simulink model "uav_airframe"  (R2023b)
settings: Solver=ode45  StartTime=0  StopTime=500  RelTol=1e-4
undefined symbols (not defined in the file): b, c, C_D, C_l, C_L, C_m, C_n, C_Q, C_T, C_Y, D, F_b, i_0, K_Q, K_V, M_b, mass, p, R_motor, S, V_max
libraries: sharedtransform x2
settings Model: Creator=Victor  LastModifiedBy=Victor
settings DataIOCC: ExternalInput=getinputstruct(report30)  InitialState=getstatestruct(report30)  SaveOutput=off  SaveTime=off
settings DebuggingCC: MaxConsecutiveZCsMsg=warning

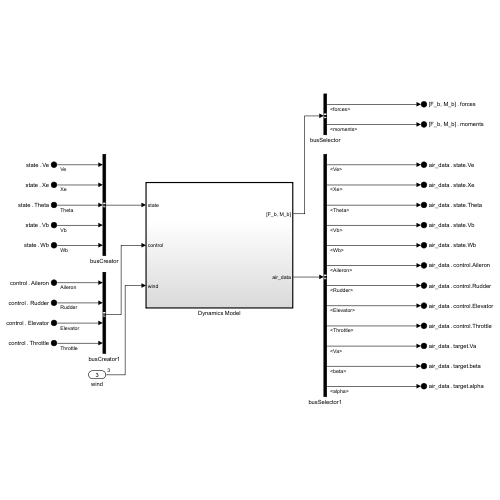
[thumbnail: Simulink's stored preview of the top-level diagram]
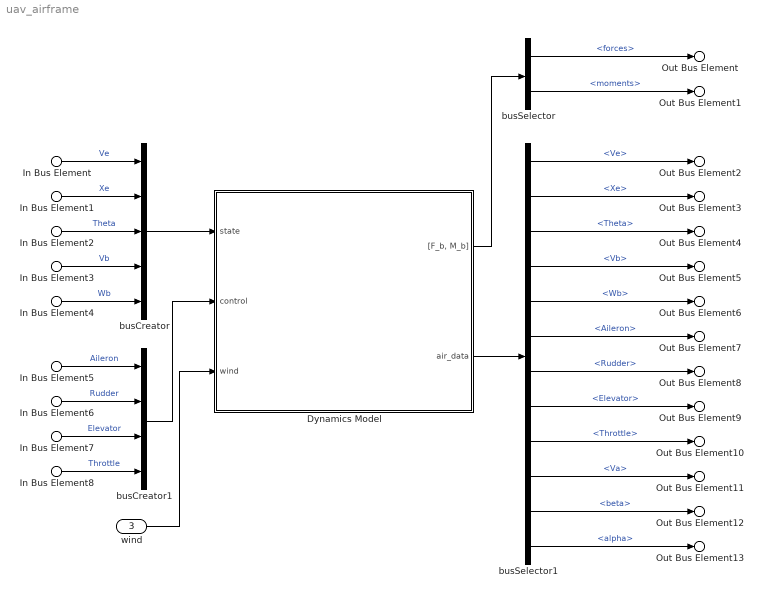
== system uav_airframe ==
  In Bus Element : Inport  PortName=state  Element=Ve
  In Bus Element1 : Inport  PortName=state  Element=Xe
  In Bus Element2 : Inport  PortName=state  Element=Theta
  In Bus Element3 : Inport  PortName=state  Element=Vb
  In Bus Element4 : Inport  PortName=state  Element=Wb
  In Bus Element5 : Inport  Port=2  PortName=control  Element=Aileron
  In Bus Element6 : Inport  Port=2  PortName=control  Element=Rudder
  In Bus Element7 : Inport  Port=2  PortName=control  Element=Elevator
  In Bus Element8 : Inport  Port=2  PortName=control  Element=Throttle
  wind : Inport  Port=3  OutDataTypeStr=double  PortDimensions=3
  Dynamics Model : Subsystem  TreatAsAtomicUnit=on
  busCreator : BusCreator  Inputs=5
  busCreator1 : BusCreator  Inputs=4
  busSelector : BusSelector  OutputSignals=forces,moments
  busSelector1 : BusSelector  OutputSignals=state.Ve,state.Xe,state.Theta,state.Vb,state.Wb,control.Aileron,control.Rudder,control.Elevator,control.Throttle,target.Va,target.beta,target.alpha
  Out Bus Element : Outport  PortName=[F_b, M_b]  Element=forces
  Out Bus Element1 : Outport  PortName=[F_b, M_b]  Element=moments
  Out Bus Element2 : Outport  Port=2  PortName=air_data  Element=state.Ve
  Out Bus Element3 : Outport  Port=2  PortName=air_data  Element=state.Xe
  Out Bus Element4 : Outport  Port=2  PortName=air_data  Element=state.Theta
  Out Bus Element5 : Outport  Port=2  PortName=air_data  Element=state.Vb
  Out Bus Element6 : Outport  Port=2  PortName=air_data  Element=state.Wb
  Out Bus Element7 : Outport  Port=2  PortName=air_data  Element=control.Aileron
  Out Bus Element8 : Outport  Port=2  PortName=air_data  Element=control.Rudder
  Out Bus Element9 : Outport  Port=2  PortName=air_data  Element=control.Elevator
  Out Bus Element10 : Outport  Port=2  PortName=air_data  Element=control.Throttle
  Out Bus Element11 : Outport  Port=2  PortName=air_data  Element=target.Va
  Out Bus Element12 : Outport  Port=2  PortName=air_data  Element=target.beta
  Out Bus Element13 : Outport  Port=2  PortName=air_data  Element=target.alpha
  wires:
  In Bus Element/1 -> busCreator/1  "Ve"
  In Bus Element1/1 -> busCreator/2  "Xe"
  In Bus Element5/1 -> busCreator1/1  "Aileron"
  In Bus Element2/1 -> busCreator/3  "Theta"
  In Bus Element6/1 -> busCreator1/2  "Rudder"
  In Bus Element3/1 -> busCreator/4  "Vb"
  In Bus Element7/1 -> busCreator1/3  "Elevator"
  In Bus Element4/1 -> busCreator/5  "Wb"
  In Bus Element8/1 -> busCreator1/4  "Throttle"
  busCreator/1 -> Dynamics Model/1(state)
  busCreator1/1 -> Dynamics Model/2(control)
  wind/1 -> Dynamics Model/3(wind)
  busSelector/2 -> Out Bus Element1/1  "<moments>"
  Dynamics Model/1("[F_b, M_b]") -> busSelector/1
  busSelector1/4 -> Out Bus Element5/1  "<Vb>"
  Dynamics Model/2(air_data) -> busSelector1/1
  busSelector/1 -> Out Bus Element/1  "<forces>"
  busSelector1/1 -> Out Bus Element2/1  "<Ve>"
  busSelector1/2 -> Out Bus Element3/1  "<Xe>"
  busSelector1/3 -> Out Bus Element4/1  "<Theta>"
  busSelector1/5 -> Out Bus Element6/1  "<Wb>"
  busSelector1/6 -> Out Bus Element7/1  "<Aileron>"
  busSelector1/7 -> Out Bus Element8/1  "<Rudder>"
  busSelector1/8 -> Out Bus Element9/1  "<Elevator>"
  busSelector1/9 -> Out Bus Element10/1  "<Throttle>"
  busSelector1/10 -> Out Bus Element11/1  "<Va>"
  busSelector1/11 -> Out Bus Element12/1  "<beta>"
  busSelector1/12 -> Out Bus Element13/1  "<alpha>"

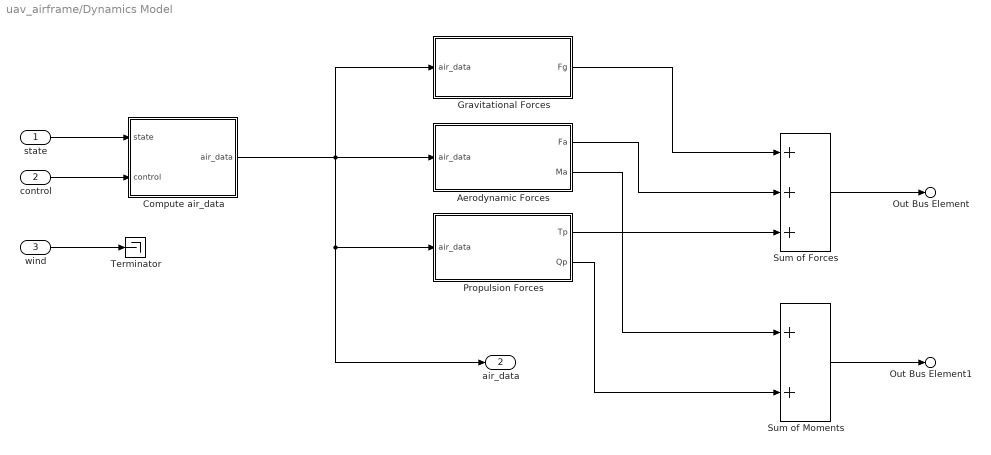
== system uav_airframe/Dynamics Model ==
  state : Inport
  control : Inport  Port=2
  wind : Inport  Port=3
  Aerodynamic Forces : Subsystem
  Compute air_data : Subsystem
  Gravitational Forces : Subsystem
  Propulsion Forces : Subsystem
  Sum of Forces : Sum  Inputs=+++
  Sum of Moments : Sum
  Terminator : Terminator
  Out Bus Element : Outport  PortName=[F_b, M_b]  Element=forces
  Out Bus Element1 : Outport  PortName=[F_b, M_b]  Element=moments
  air_data : Outport  Port=2
  wires:
  Propulsion Forces/2(Qp) -> Sum of Moments/2
  Propulsion Forces/1(Tp) -> Sum of Forces/3
  Compute air_data/1(air_data) -> Aerodynamic Forces/1(air_data), Gravitational Forces/1(air_data), air_data/1, Propulsion Forces/1(air_data)
  control/1 -> Compute air_data/2(control)
  state/1 -> Compute air_data/1(state)
  wind/1 -> Terminator/1
  Sum of Forces/1 -> Out Bus Element/1
  Sum of Moments/1 -> Out Bus Element1/1
  Gravitational Forces/1(Fg) -> Sum of Forces/1
  Aerodynamic Forces/1(Fa) -> Sum of Forces/2
  Aerodynamic Forces/2(Ma) -> Sum of Moments/1

== system uav_airframe/Dynamics Model/Aerodynamic Forces ==
  air_data : Inport
  Add : Sum
  Add1 : Sum
  Lateral Forces : Subsystem
  Longitudinal Forces : Subsystem
  Fa : Outport
  Ma : Outport  Port=2
  wires:
  air_data/1 -> Lateral Forces/1(air_data), Longitudinal Forces/1(air_data)
  Lateral Forces/1(faL_b) -> Add/1
  Longitudinal Forces/1(fa_b) -> Add/2
  Add/1 -> Fa/1
  Lateral Forces/2(MaL_b) -> Add1/1
  Longitudinal Forces/2(Ma_b) -> Add1/2
  Add1/1 -> Ma/1

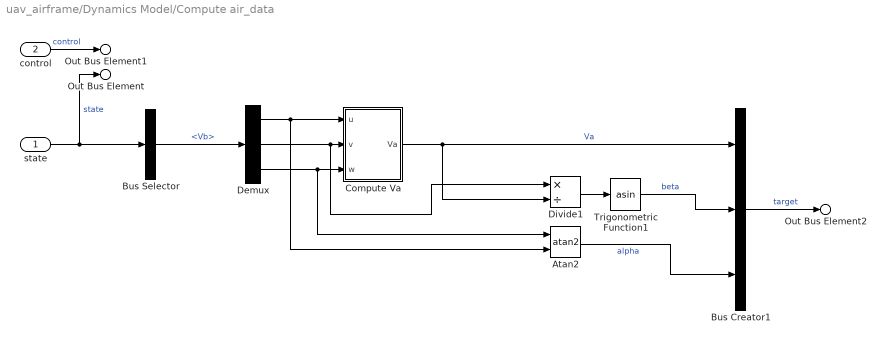
== system uav_airframe/Dynamics Model/Compute air_data ==
  state : Inport
  control : Inport  Port=2
  Atan2 : Trigonometry  Operator=atan2
  Bus Creator1 : BusCreator  Inputs=3
  Bus Selector : BusSelector  OutputSignals=Vb
  Compute Va : Subsystem
  Demux : Demux  Outputs=3
  Divide1 : Product  Inputs=*/
  Trigonometric Function1 : Trigonometry  Operator=asin
  Out Bus Element : Outport  PortName=air_data  Element=state
  Out Bus Element1 : Outport  PortName=air_data  Element=control
  Out Bus Element2 : Outport  PortName=air_data  Element=target
  wires:
  Demux/3 -> Atan2/1, Compute Va/3(w)
  Bus Selector/1 -> Demux/1  "<Vb>"
  control/1 -> Out Bus Element1/1  "control"
  Bus Creator1/1 -> Out Bus Element2/1  "target"
  Demux/1 -> Atan2/2, Compute Va/1(u)
  Demux/2 -> Compute Va/2(v), Divide1/1
  Atan2/1 -> Bus Creator1/3  "alpha"
  Compute Va/1(Va) -> Bus Creator1/1, Divide1/2  "Va"
  Divide1/1 -> Trigonometric Function1/1
  Trigonometric Function1/1 -> Bus Creator1/2  "beta"
  state/1 -> Bus Selector/1, Out Bus Element/1  "state"

== system uav_airframe/Dynamics Model/Gravitational Forces ==
  air_data : Inport
  Bus Selector : BusSelector  OutputSignals=state.Theta
  Gravity : Gain  Gain=9.81
  Mass : Constant  Value=mass
  NED : Concatenate  NumInputs=3
  Vehicle-frame to Body-frame : Subsystem
  Zero : Constant  Value=0  OutDataTypeStr=Inherit: Inherit via back propagation
  Fg : Outport
  wires:
  Bus Selector/1 -> Vehicle-frame to Body-frame/1(Theta)  "<Theta>"
  air_data/1 -> Bus Selector/1
  Vehicle-frame to Body-frame/1(Fg_b) -> Fg/1
  NED/1 -> Vehicle-frame to Body-frame/2(Fg_v)  "Fg_v"
  Zero/1 -> NED/2, NED/1
  Gravity/1 -> NED/3
  Mass/1 -> Gravity/1

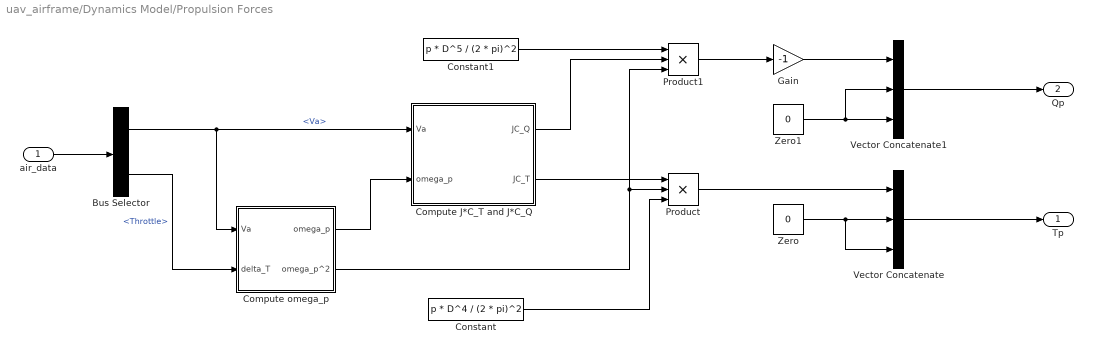
== system uav_airframe/Dynamics Model/Propulsion Forces ==
  air_data : Inport
  Bus Selector : BusSelector  OutputSignals=target.Va,control.Throttle
  Compute J*C_T and J*C_Q : Subsystem
  Compute omega_p : Subsystem
  Constant : Constant  Value=p * D^4 / (2 * pi)^2
  Constant1 : Constant  Value=p * D^5 / (2 * pi)^2
  Gain : Gain  Gain=-1
  Product : Product  Inputs=3
  Product1 : Product  Inputs=3
  Vector Concatenate : Concatenate  NumInputs=3
  Vector Concatenate1 : Concatenate  NumInputs=3
  Zero : Constant  Value=0  OutDataTypeStr=Inherit: Inherit via back propagation
  Zero1 : Constant  Value=0  OutDataTypeStr=Inherit: Inherit via back propagation
  Tp : Outport
  Qp : Outport  Port=2
  wires:
  Constant/1 -> Product/3
  Compute J*C_T and J*C_Q/1(JC_Q) -> Product1/2
  Bus Selector/2 -> Compute omega_p/2(delta_T)  "<Throttle>"
  Constant1/1 -> Product1/1
  Compute J*C_T and J*C_Q/2(JC_T) -> Product/1
  Bus Selector/1 -> Compute omega_p/1(Va), Compute J*C_T and J*C_Q/1(Va)  "<Va>"
  Compute omega_p/1(omega_p) -> Compute J*C_T and J*C_Q/2(omega_p)
  Compute omega_p/2(omega_p^2) -> Product1/3, Product/2
  Product1/1 -> Gain/1
  Product/1 -> Vector Concatenate/1
  air_data/1 -> Bus Selector/1
  Gain/1 -> Vector Concatenate1/1
  Vector Concatenate1/1 -> Qp/1
  Zero1/1 -> Vector Concatenate1/3, Vector Concatenate1/2
  Vector Concatenate/1 -> Tp/1
  Zero/1 -> Vector Concatenate/3, Vector Concatenate/2

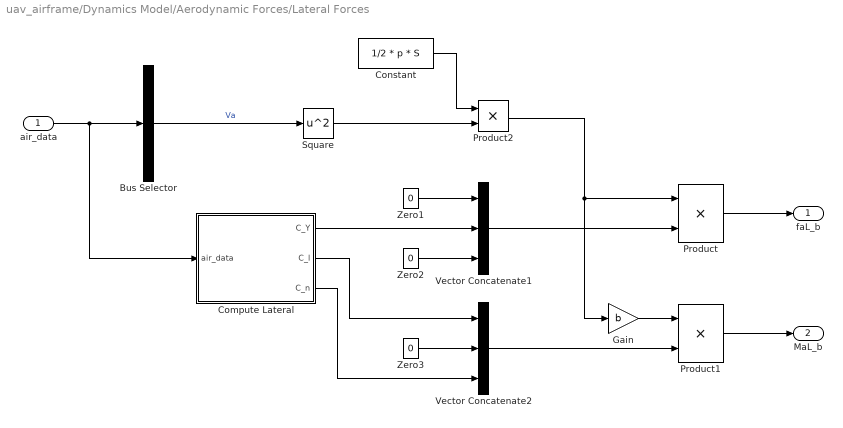
== system uav_airframe/Dynamics Model/Aerodynamic Forces/Lateral Forces ==
  air_data : Inport
  Bus Selector : BusSelector  OutputSignals=target.Va  OutputAsBus=on
  Compute Lateral : Subsystem
  Constant : Constant  Value=1/2 * p * S
  Gain : Gain  Gain=b
  Product : Product
  Product1 : Product
  Product2 : Product
  Square : Math  Operator=square
  Vector Concatenate1 : Concatenate  NumInputs=3
  Vector Concatenate2 : Concatenate  NumInputs=3
  Zero1 : Constant  Value=0  OutDataTypeStr=Inherit: Inherit via back propagation
  Zero2 : Constant  Value=0  OutDataTypeStr=Inherit: Inherit via back propagation
  Zero3 : Constant  Value=0  OutDataTypeStr=Inherit: Inherit via back propagation
  faL_b : Outport
  MaL_b : Outport  Port=2
  wires:
  Gain/1 -> Product1/1
  Vector Concatenate2/1 -> Product1/2
  Vector Concatenate1/1 -> Product/2
  Product2/1 -> Product/1, Gain/1
  Constant/1 -> Product2/1
  Square/1 -> Product2/2
  Product1/1 -> MaL_b/1
  Zero3/1 -> Vector Concatenate2/2
  Compute Lateral/2(C_l) -> Vector Concatenate2/1
  Compute Lateral/3(C_n) -> Vector Concatenate2/3
  Compute Lateral/1(C_Y) -> Vector Concatenate1/2
  Zero2/1 -> Vector Concatenate1/3
  Zero1/1 -> Vector Concatenate1/1
  air_data/1 -> Bus Selector/1, Compute Lateral/1(air_data)
  Product/1 -> faL_b/1
  Bus Selector/1 -> Square/1  "Va"

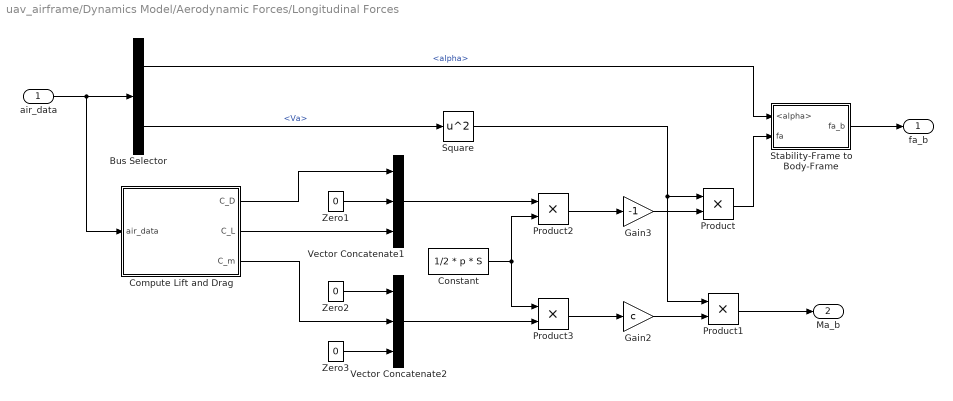
== system uav_airframe/Dynamics Model/Aerodynamic Forces/Longitudinal Forces ==
  air_data : Inport
  Bus Selector : BusSelector  OutputSignals=target.alpha,target.Va
  Compute Lift and Drag : Subsystem
  Constant : Constant  Value=1/2 * p * S
  Gain2 : Gain  Gain=c
  Gain3 : Gain  Gain=-1
  Product{,1..3} (4 alike) : Product
  Square : Math  Operator=square
  Stability-Frame to Body-Frame : Subsystem
  Vector Concatenate1 : Concatenate  NumInputs=3
  Vector Concatenate2 : Concatenate  NumInputs=3
  Zero1 : Constant  Value=0  OutDataTypeStr=Inherit: Inherit via back propagation
  Zero2 : Constant  Value=0  OutDataTypeStr=Inherit: Inherit via back propagation
  Zero3 : Constant  Value=0  OutDataTypeStr=Inherit: Inherit via back propagation
  fa_b : Outport
  Ma_b : Outport  Port=2
  wires:
  Product/1 -> Stability-Frame to Body-Frame/2(fa)
  Square/1 -> Product/1, Product1/1
  Gain3/1 -> Product/2
  Gain2/1 -> Product1/2
  Product3/1 -> Gain2/1
  Product2/1 -> Gain3/1
  Constant/1 -> Product3/1, Product2/2
  Zero2/1 -> Vector Concatenate2/1
  Stability-Frame to Body-Frame/1(fa_b) -> fa_b/1
  Bus Selector/1 -> Stability-Frame to Body-Frame/1(<alpha>)  "<alpha>"
  Bus Selector/2 -> Square/1  "<Va>"
  Product1/1 -> Ma_b/1
  Compute Lift and Drag/3(C_m) -> Vector Concatenate2/2
  Zero3/1 -> Vector Concatenate2/3
  Vector Concatenate2/1 -> Product3/2
  Compute Lift and Drag/2(C_L) -> Vector Concatenate1/3
  Compute Lift and Drag/1(C_D) -> Vector Concatenate1/1
  Zero1/1 -> Vector Concatenate1/2
  Vector Concatenate1/1 -> Product2/1
  air_data/1 -> Compute Lift and Drag/1(air_data), Bus Selector/1

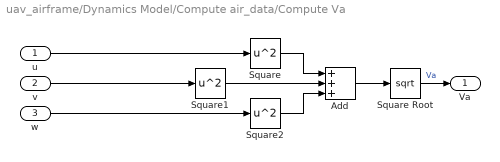
== system uav_airframe/Dynamics Model/Compute air_data/Compute Va ==
  u : Inport
  v : Inport  Port=2
  w : Inport  Port=3
  Add : Sum  Inputs=+++
  Square : Math  Operator=square
  Square Root : Sqrt
  Square1 : Math  Operator=square
  Square2 : Math  Operator=square
  Va : Outport
  wires:
  Square Root/1 -> Va/1  "Va"
  v/1 -> Square1/1
  w/1 -> Square2/1
  u/1 -> Square/1
  Square1/1 -> Add/2
  Add/1 -> Square Root/1
  Square/1 -> Add/1
  Square2/1 -> Add/3

== system uav_airframe/Dynamics Model/Gravitational Forces/Vehicle-frame to Body-frame ==
  Theta : Inport
  Fg_v : Inport  Port=2
  Matrix Multiply : Product  Multiplication=Matrix(*)
  R^v_b : sharedtransform/Rotation Angles to Direction Cosine Matrix  rotationOrder=ZYX  aMode=aMode
  Reshape : Reshape  OutputDimensionality=Column vector (2-D)
  Reshape1 : Reshape
  Selector : Selector  InputPortWidth=3  IndexOptions=Index vector (dialog)  Indices=[3 2 1]  OutputSizes=1
  Fg_b : Outport
  wires:
  Reshape1/1 -> Fg_b/1
  Reshape/1 -> Matrix Multiply/2
  Fg_v/1 -> Reshape/1
  R^v_b/1 -> Matrix Multiply/1
  Selector/1 -> R^v_b/1
  Theta/1 -> Selector/1
  Matrix Multiply/1 -> Reshape1/1

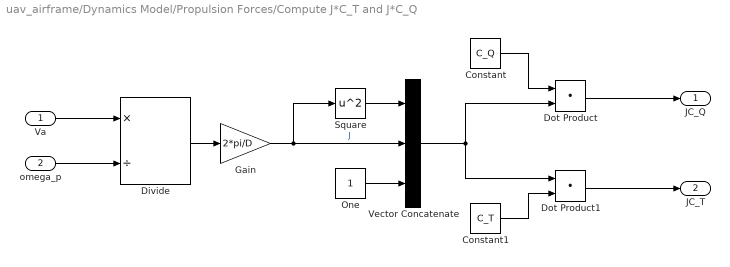
== system uav_airframe/Dynamics Model/Propulsion Forces/Compute J*C_T and J*C_Q ==
  Va : Inport
  omega_p : Inport  Port=2
  Constant : Constant  Value=C_Q
  Constant1 : Constant  Value=C_T
  Divide : Product  Inputs=*/
  Dot Product : DotProduct  OutDataTypeStr=Inherit: Inherit via internal rule
  Dot Product1 : DotProduct  OutDataTypeStr=Inherit: Inherit via internal rule
  Gain : Gain  Gain=2*pi/D
  One : Constant  OutDataTypeStr=Inherit: Inherit via back propagation
  Square : Math  Operator=square
  Vector Concatenate : Concatenate  NumInputs=3
  JC_Q : Outport
  JC_T : Outport  Port=2
  wires:
  Dot Product/1 -> JC_Q/1
  Dot Product1/1 -> JC_T/1
  Constant1/1 -> Dot Product1/2
  Vector Concatenate/1 -> Dot Product/2, Dot Product1/1
  Constant/1 -> Dot Product/1
  One/1 -> Vector Concatenate/3
  Square/1 -> Vector Concatenate/1
  Gain/1 -> Vector Concatenate/2, Square/1  "J"
  Divide/1 -> Gain/1
  omega_p/1 -> Divide/2
  Va/1 -> Divide/1

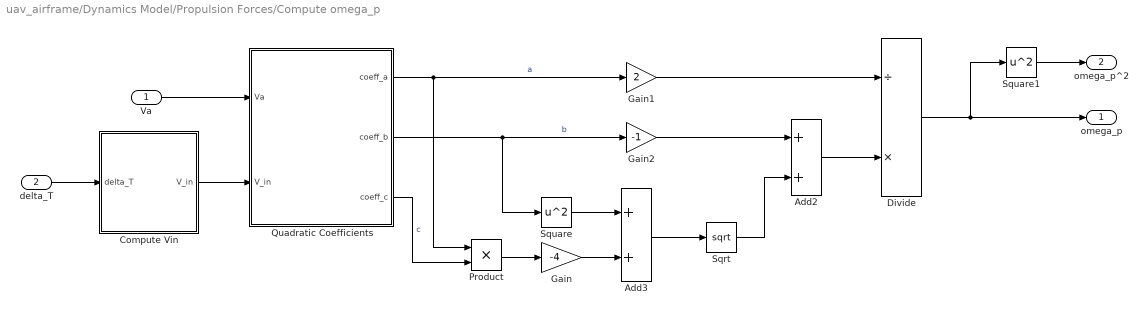
== system uav_airframe/Dynamics Model/Propulsion Forces/Compute omega_p ==
  Va : Inport
  delta_T : Inport  Port=2
  Add2 : Sum
  Add3 : Sum
  Compute Vin : Subsystem
  Divide : Product  Inputs=/*
  Gain : Gain  Gain=-4
  Gain1 : Gain  Gain=2
  Gain2 : Gain  Gain=-1
  Product : Product
  Quadratic Coefficients : Subsystem
  Sqrt : Sqrt
  Square : Math  Operator=square
  Square1 : Math  Operator=square
  omega_p : Outport
  omega_p^2 : Outport  Port=2
  wires:
  Add2/1 -> Divide/2
  Quadratic Coefficients/3(coeff_c) -> Product/2  "c"
  Gain/1 -> Add3/2
  Square/1 -> Add3/1
  Add3/1 -> Sqrt/1
  Sqrt/1 -> Add2/2
  Gain2/1 -> Add2/1
  Quadratic Coefficients/2(coeff_b) -> Gain2/1, Square/1  "b"
  Gain1/1 -> Divide/1
  Quadratic Coefficients/1(coeff_a) -> Gain1/1, Product/1  "a"
  Square1/1 -> omega_p^2/1
  Compute Vin/1(V_in) -> Quadratic Coefficients/2(V_in)
  Va/1 -> Quadratic Coefficients/1(Va)
  Divide/1 -> Square1/1, omega_p/1
  Product/1 -> Gain/1
  delta_T/1 -> Compute Vin/1(delta_T)

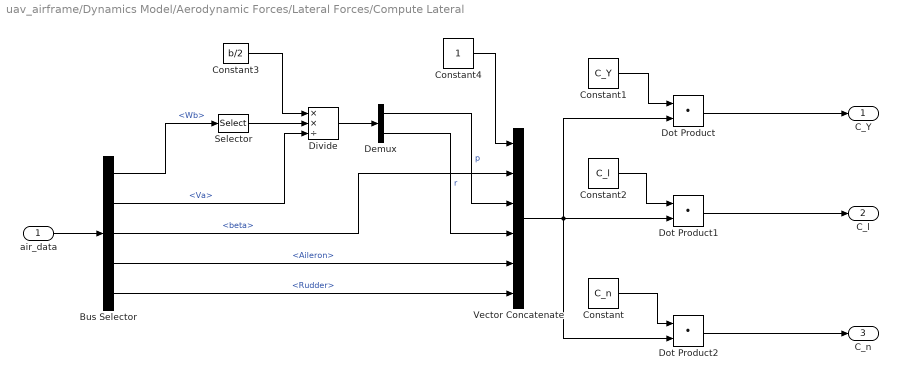
== system uav_airframe/Dynamics Model/Aerodynamic Forces/Lateral Forces/Compute Lateral ==
  air_data : Inport
  Bus Selector : BusSelector  OutputSignals=state.Wb,target.Va,target.beta,control.Aileron,control.Rudder
  Constant : Constant  Value=C_n
  Constant1 : Constant  Value=C_Y
  Constant2 : Constant  Value=C_l
  Constant3 : Constant  Value=b/2
  Constant4 : Constant
  Demux : Demux  Outputs=2
  Divide : Product  Inputs=**/
  Dot Product : DotProduct  OutDataTypeStr=Inherit: Inherit via internal rule
  Dot Product1 : DotProduct  OutDataTypeStr=Inherit: Inherit via internal rule
  Dot Product2 : DotProduct  OutDataTypeStr=Inherit: Inherit via internal rule
  Selector : Selector  InputPortWidth=3  IndexOptions=Index vector (dialog)  Indices=[1 3]  OutputSizes=1
  Vector Concatenate : Concatenate  NumInputs=6
  C_Y : Outport
  C_l : Outport  Port=2
  C_n : Outport  Port=3
  wires:
  Constant3/1 -> Divide/1
  Bus Selector/5 -> Vector Concatenate/6  "<Rudder>"
  Bus Selector/4 -> Vector Concatenate/5  "<Aileron>"
  Bus Selector/3 -> Vector Concatenate/2  "<beta>"
  Bus Selector/2 -> Divide/3  "<Va>"
  Bus Selector/1 -> Selector/1  "<Wb>"
  Constant/1 -> Dot Product2/1
  Divide/1 -> Demux/1
  Demux/2 -> Vector Concatenate/4  "r"
  Demux/1 -> Vector Concatenate/3  "p"
  Constant4/1 -> Vector Concatenate/1
  Selector/1 -> Divide/2
  Dot Product2/1 -> C_n/1
  Dot Product1/1 -> C_l/1
  Dot Product/1 -> C_Y/1
  Constant2/1 -> Dot Product1/1
  Vector Concatenate/1 -> Dot Product/2, Dot Product1/2, Dot Product2/2
  Constant1/1 -> Dot Product/1
  air_data/1 -> Bus Selector/1

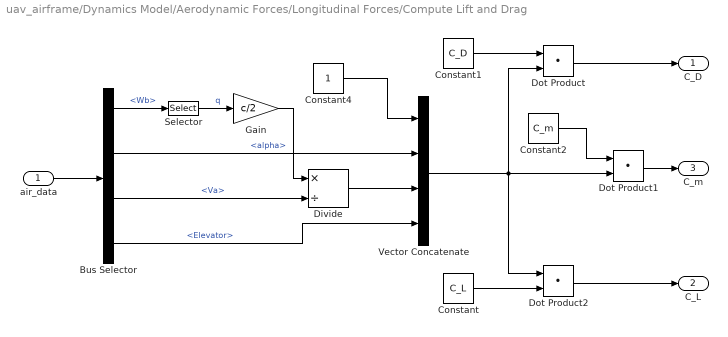
== system uav_airframe/Dynamics Model/Aerodynamic Forces/Longitudinal Forces/Compute Lift and Drag ==
  air_data : Inport
  Bus Selector : BusSelector  OutputSignals=state.Wb,target.alpha,target.Va,control.Elevator
  Constant : Constant  Value=C_L
  Constant1 : Constant  Value=C_D
  Constant2 : Constant  Value=C_m
  Constant4 : Constant
  Divide : Product  Inputs=*/
  Dot Product : DotProduct  OutDataTypeStr=Inherit: Inherit via internal rule
  Dot Product1 : DotProduct  OutDataTypeStr=Inherit: Inherit via internal rule
  Dot Product2 : DotProduct  OutDataTypeStr=Inherit: Inherit via internal rule
  Gain : Gain  Gain=c/2
  Selector : Selector  InputPortWidth=3  IndexOptions=Index vector (dialog)  Indices=[2]  OutputSizes=1
  Vector Concatenate : Concatenate  NumInputs=4
  C_D : Outport
  C_L : Outport  Port=2
  C_m : Outport  Port=3
  wires:
  Bus Selector/1 -> Selector/1  "<Wb>"
  Selector/1 -> Gain/1  "q"
  Dot Product2/1 -> C_L/1
  Dot Product1/1 -> C_m/1
  Dot Product/1 -> C_D/1
  Constant2/1 -> Dot Product1/1
  Constant/1 -> Dot Product2/2
  Vector Concatenate/1 -> Dot Product/2, Dot Product1/2, Dot Product2/1
  Constant1/1 -> Dot Product/1
  Bus Selector/4 -> Vector Concatenate/4  "<Elevator>"
  Divide/1 -> Vector Concatenate/3
  Gain/1 -> Divide/1
  Bus Selector/3 -> Divide/2  "<Va>"
  Bus Selector/2 -> Vector Concatenate/2  "<alpha>"
  air_data/1 -> Bus Selector/1
  Constant4/1 -> Vector Concatenate/1

== system uav_airframe/Dynamics Model/Aerodynamic Forces/Longitudinal Forces/Stability-Frame to Body-Frame ==
  <alpha> : Inport
  fa : Inport  Port=2
  Rotation Angles to Direction Cosine Matrix : sharedtransform/Rotation Angles to Direction Cosine Matrix  rotationOrder=ZYX  aMode=aMode
  Stability-Frame to Body-Frame : Product  Multiplication=Matrix(*)
  Vector Concatenate : Concatenate  NumInputs=3
  Zero : Constant  Value=0  OutDataTypeStr=Inherit: Inherit via back propagation
  fa_b : Outport
  wires:
  Stability-Frame to Body-Frame/1 -> fa_b/1
  fa/1 -> Stability-Frame to Body-Frame/2
  Vector Concatenate/1 -> Rotation Angles to Direction Cosine Matrix/1  "[0, a, 0]"
  Zero/1 -> Vector Concatenate/1, Vector Concatenate/3
  Rotation Angles to Direction Cosine Matrix/1 -> Stability-Frame to Body-Frame/1  "R^s_b"
  <alpha>/1 -> Vector Concatenate/2

== system uav_airframe/Dynamics Model/Propulsion Forces/Compute omega_p/Compute Vin ==
  delta_T : Inport
  Product : Product
  V_max : Constant  Value=V_max
  V_in : Outport
  wires:
  delta_T/1 -> Product/1
  Product/1 -> V_in/1
  V_max/1 -> Product/2

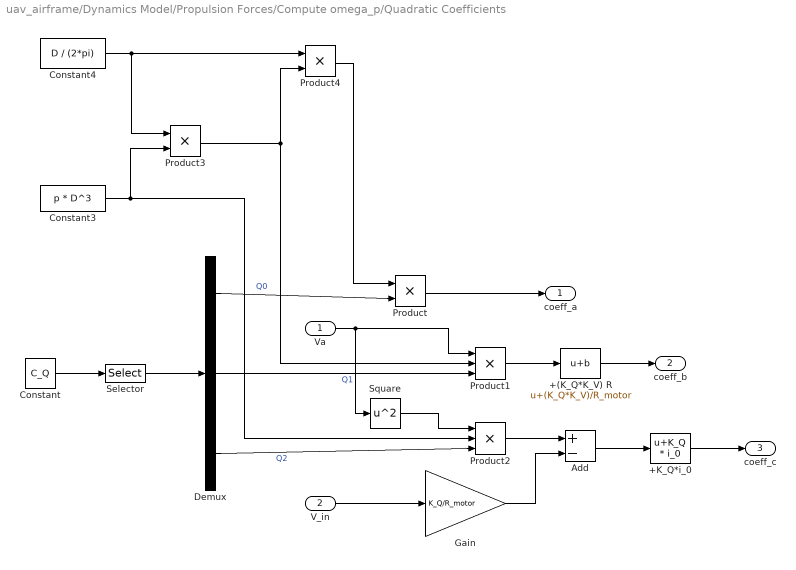
== system uav_airframe/Dynamics Model/Propulsion Forces/Compute omega_p/Quadratic Coefficients ==
  Va : Inport
  V_in : Inport  Port=2
  +(K_Q*K_V) R : Bias  Bias=(K_Q*K_V)/R_motor  SaturateOnIntegerOverflow=off
  +K_Q*i_0 : Bias  Bias=K_Q * i_0  SaturateOnIntegerOverflow=off
  Add : Sum  Inputs=+-
  Constant : Constant  Value=C_Q
  Constant3 : Constant  Value=p * D^3
  Constant4 : Constant  Value=D / (2*pi)
  Demux : Demux  Outputs=3
  Gain : Gain  Gain=K_Q/R_motor
  Product : Product
  Product1 : Product  Inputs=3
  Product2 : Product  Inputs=3
  Product3 : Product
  Product4 : Product
  Selector : Selector  InputPortWidth=3  IndexOptions=Index vector (dialog)  Indices=[3 2 1]  OutputSizes=1
  Square : Math  Operator=square
  coeff_a : Outport
  coeff_b : Outport  Port=2
  coeff_c : Outport  Port=3
  wires:
  +K_Q*i_0/1 -> coeff_c/1
  Add/1 -> +K_Q*i_0/1
  Gain/1 -> Add/2
  V_in/1 -> Gain/1
  Product2/1 -> Add/1
  Square/1 -> Product2/1
  +(K_Q*K_V) R/1 -> coeff_b/1
  Product1/1 -> +(K_Q*K_V) R/1
  Va/1 -> Product1/1, Square/1
  Product/1 -> coeff_a/1
  Product4/1 -> Product/1
  Demux/3 -> Product2/3  "Q2"
  Demux/2 -> Product1/3  "Q1"
  Demux/1 -> Product/2  "Q0"
  Selector/1 -> Demux/1
  Constant/1 -> Selector/1
  Product3/1 -> Product4/2, Product1/2
  Constant4/1 -> Product3/1, Product4/1
  Constant3/1 -> Product3/2, Product2/2
